simulink model "regulacion_nominal_modelo_lineal"  (R2021a)
settings: Solver=VariableStepAuto  StartTime=0.0  StopTime=15  RelTol=1e-3
settings Model: Creator=jmata  LastModifiedBy=jmata

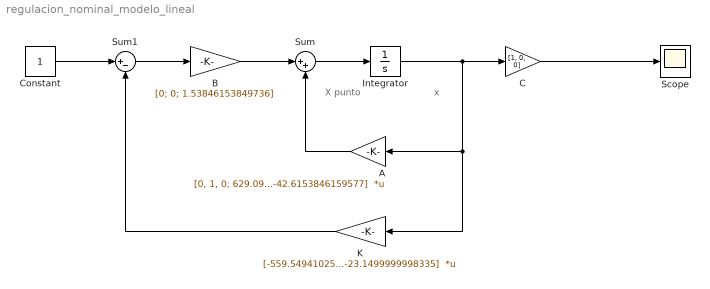
== system regulacion_nominal_modelo_lineal ==
  note: x
  note: X punto
  "A " : Gain  Gain="[0, 1, 0; 629.09300494194, 0, -5.12711320724338;  0, 0, -42.6153846159577]"  Multiplication=Matrix(K*u)
  "B " : Gain  Gain=[0; 0; 1.53846153849736]
  "C " : Gain  Gain=[1, 0, 0]
  Constant : Constant
  Integrator : Integrator
  K : Gain  Gain=[-559.549410259276, -81.2758440000597, -23.1499999998335]  Multiplication=Matrix(K*u)
  Scope : Scope
  Sum : Sum  Inputs=|++
  Sum1 : Sum  Inputs=|+-
  wires:
  "A "/1 -> Sum/2
  "B "/1 -> Sum/1
  Sum/1 -> Integrator/1
  Integrator/1 -> K/1, "A "/1, "C "/1
  "C "/1 -> Scope/1
  Constant/1 -> Sum1/1
  Sum1/1 -> "B "/1
  K/1 -> Sum1/2
